simulink model "Q2sim"  (R2018a)
settings: Solver=VariableStepAuto  StartTime=0.0  StopTime=40  RelTol=1e-3
values from neighbouring files (symbols this model uses):
  A = [0 1 0 0 ;0 -2.2626 -0.3962 0.0082; 0 0 0 1;0 3.5649 16.0655 -0.3324]    [Q1.m]    (also in Q2.m; Q3.m; Q4.m)
  B = [0; 0.2263; 0; -0.3565]    [Q1.m]    (also in Q2.m; Q3.m; Q4.m)
  C = eye(4,4)    [Q1.m]    (also in Q2.m; Q3.m; Q4.m = [1 0 0 0])
  D = [0 0 0 0]'    [Q1.m]    (also in Q2.m; Q3.m; Q4.m = 0)
  K = acker(Abar,Bbar,[-1 -2 -3 -4 -5])    [Q2.m]    (also in Q3.m = acker(A,B,[-1 -2 -3 -4]); Q4.m = acker(A,B,[-1 -2 -3 -4]))
settings Model: Creator=Siavash  LastModifiedBy=Siavash

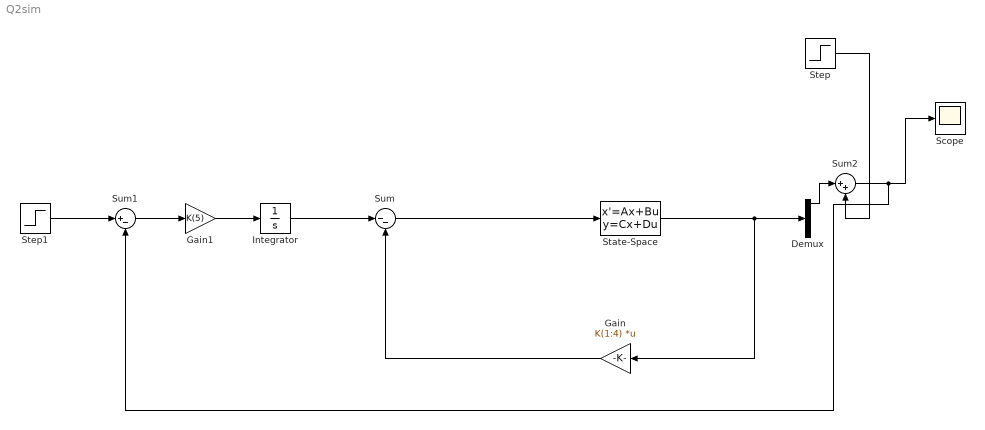
== system Q2sim ==
  Demux : Demux
  Gain : Gain  Gain=K(1:4)  Multiplication=Matrix(K*u)
  Gain1 : Gain  Gain=K(5)
  Integrator : Integrator
  Scope : Scope
  State-Space : StateSpace  A=A  B=B  C=C  D=D  InitialCondition=0
  Step : Step  Time=10  After=0.3  SampleTime=0
  Step1 : Step  Time=0  SampleTime=0
  Sum : Sum  Inputs=|--
  Sum1 : Sum  Inputs=|+-
  Sum2 : Sum  Inputs=|++
  wires:
  Demux/1 -> Sum2/1
  Gain/1 -> Sum/2
  Sum/1 -> State-Space/1
  Integrator/1 -> Sum/1
  Step1/1 -> Sum1/1
  Sum1/1 -> Gain1/1
  Gain1/1 -> Integrator/1
  State-Space/1 -> Gain/1, Demux/1
  Sum2/1 -> Sum1/2, Scope/1
  Step/1 -> Sum2/2
